simulink model "COM_ViconController_x4morf_quat"  (Simulink 8.6)
settings: Solver=FixedStepDiscrete  StartTime=0.0  StopTime=inf  FixedStep=ComMinSampleTime  RelTol=1e-3
values from neighbouring files (symbols this model uses):
  a_PWM = (MaxThrottle-MinThrottle)/(omega_r_max-omega_r_min)    [RobotParameters.m]
  b_PWM = MinThrottle - a_PWM*omega_r_min    [RobotParameters.m]
  BiasAcc = [0.52334832668 1 0]    [AccCalib_Transformation_GusRobot.mat]
  ComMinSampleTime = 1/400    (= 0.0025)    [init_ViconController_x4morf_quat.m]
  g = 9.81    [RobotParameters.m]    (also in init_ViconController_x4morf_quat.m)
  iGamma = inv(Gamma)    [RobotParameters.m]
  LandingHeight = 0.06    [init_ViconController_x4morf_quat.m]
  m = 0.376    [RobotParameters.m]
  MaxThrottle = 2000    [RobotParameters.m]
  MinThrottle = 1100    [RobotParameters.m]
  Tacc = [1  0  0; 0  1  0; 0  0  1]    [AccCalib_Transformation_GusRobot.mat]
  Tmax = .160    (= 0.16)    [RobotParameters.m]
  Tmin = .02    (= 0.02)    [RobotParameters.m]
  Velocity_0 = [Vx_0 Vy_0 Vz_0]    [RobotParameters.m]
undefined symbols (not defined in the file or in its folder): DiscIntNeverNeededParam, Gumstix, MPU6050, UAVstruct
undefined symbols (not defined in the file): AccMax, AccMin, b_est0, PositionMax, PositionMin, SpeedMax, SpeedMin, Ts_AttitudeLoop, Ts_Wifi
libraries: simulink x16, simulink_extras x6
(part 1 of 2)
settings Model: Creator=Kjenab  LastModifiedBy=valentin_riviere  ExtModeTrigDuration=10000
settings SolverCC: PositivePriorityOrder=on
settings DataIOCC: SaveFormat=StructureWithTime
settings OptimizationCC: InitFltsAndDblsToZero=on  OptimizeModelRefInitCode=on  LifeSpan=Inf  SimCompilerOptimization=on
settings DebuggingCC: SaveWithParameterizedLinksMsg=none  UnderspecifiedInitializationDetection=Simplified  MergeDetectMultiDrivingBlocksExec=error  FcnCallInpInsideContextMsg=UseLocalSettings
settings HardwareCC: ProdHWDeviceType=Generic->Unspecified (assume 32-bit Generic)
settings RTWCC: SystemTargetFile=ert.tlc  GenCodeOnly=on  GenerateMakefile=off  TemplateMakefile=ert_default_tmf  PostCodeGenCommand=packNGo(buildInfo, {'packType' 'hierarchical'})  Description=Embedded Coder  RTWCompilerOptimization=on
settings CodeAppCC: IgnoreCustomStorageClasses=off  CustomSymbolStrType=$N$R$M  InternalIdentifier=Classic
settings ERTTargetCC: MultiwordLength=2048  GenerateSampleERTMain=on  ERTCustomFileTemplate=example_file_process.tlc  ConvertIfToSwitch=off  SuppressUnreachableDefaultCases=off

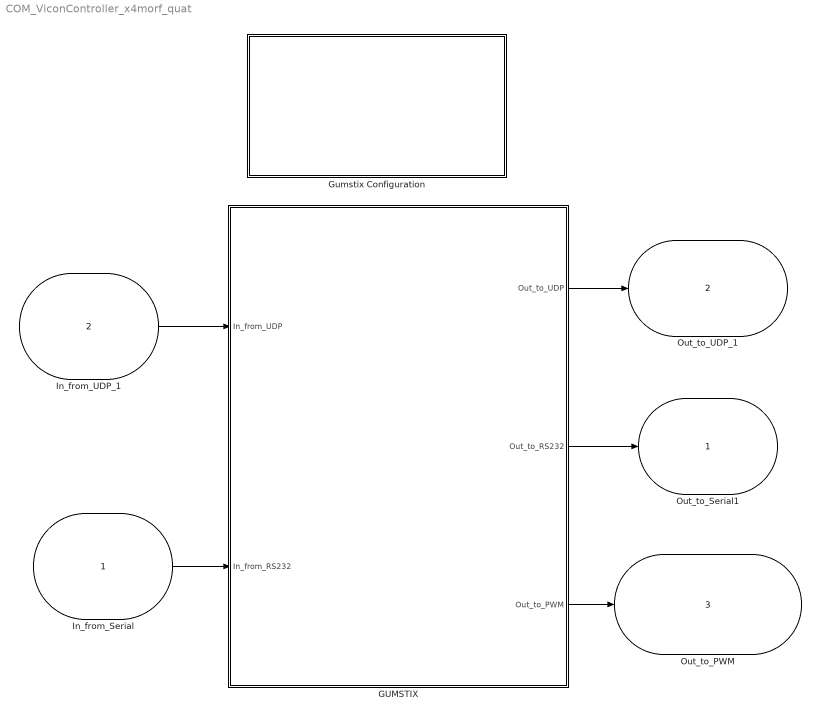
== system COM_ViconController_x4morf_quat ==
  In_from_Serial : Inport  OutDataTypeStr=int16  PortDimensions=Gumstix.RS232.Reception(1).NbData  SampleTime=Gumstix.RS232.Reception(1).SampleTime  mask{RS232_NbData=11, RS232_DataType=int16, RS232_Port=/dev/ttyO0, RS232_BaudRate=115200, RS232_SampleTime=Ts_AttitudeLoop, RS232_BlockingReception=OFF (try to read the n data), RS232_BlockingTimeOut=0.00022, RS232_StreamHeaderReception=1 byte, RS232_StreamHeaderValue=170, RS232_StartProtocol=SendStart -> WaitStart, RS232_StartTimeOut=100, RS232_StartStream=START, RS232_StopProtocol=None, RS232_StopTimeOut=100, RS232_StopStream=STOP}
      mask prompts: RS232_NbData "Number of Received Data"; RS232_DataType "RS232 Data Type"; RS232_Port "Serial Port"; RS232_BaudRate "BaudRate"; RS232_SampleTime "Reception Sample Time [s]"; RS232_BlockingReception "Blocking Reception"; RS232_BlockingTimeOut "Blocking Time Out [s]"; RS232_StreamHeaderReception "Stream Header"; RS232_StreamHeaderValue "Stream header value [0-255]"; RS232_StartProtocol "START Protocols"; RS232_StartTimeOut "Start Stream Waiting TimeOut [ms]"; RS232_StartStream "Start Message"; RS232_StopProtocol "STOP Protocols"; RS232_StopTimeOut "Stop Stream Waiting TimeOut [ms]"; RS232_StopStream "Stop Message"
      mask init:
      | for i=1:1:15
      |     ProcessRS232InportMask_COM(gcb, i);
      | end
      mask Callback RS232_NbData: ProcessRS232InportMask_COM(gcb, 1);
      mask TypeOptions RS232_DataType: double64 | float32 | int32 | unsigned int32 | int16 | unsigned int16 | char8 | unsigned char8
      mask Callback RS232_DataType: ProcessRS232InportMask_COM(gcb, 2);
      mask TypeOptions RS232_Port: /dev/ttyO0 | /dev/ttyO1 | /dev/ttyO2 | /dev/ttyO3 | /dev/ttyO4 | /dev/ttyO5 | /dev/ttyO6 | /dev/ttyO7 | /dev/ttyO8 | /dev/ttyO9 | /dev/ttyO10 | /dev/ttyO11 | /dev/ttyO12 | /dev/ttyO13 | /dev/ttyO14 | /dev/ttyO15 | /dev/ttyUSB0 | /dev/ttyUSB1
      mask Callback RS232_Port: ProcessRS232InportMask_COM(gcb, 3);
      mask TypeOptions RS232_BaudRate: 50 | 75 | 110 | 134 | 150 | 200 | 300 | 600 | 1200 | 1800 | 2400 | 4800 | 9600 | 19200 | 38400 | 57600 | 115200 | 230400 | 460800 | 576000 | 921600 | 1000000 | 1152000 | 1500000 | 2000000 | 2500000 | 3000000 | 3500000 | 4000000
      mask Callback RS232_BaudRate: ProcessRS232InportMask_COM(gcb, 4);
      mask Callback RS232_SampleTime: ProcessRS232InportMask_COM(gcb, 5);
      mask TypeOptions RS232_BlockingReception: ON (wait the n data) | OFF (try to read the n data)
      mask Callback RS232_BlockingReception: ProcessRS232InportMask_COM(gcb, 6);
      mask Callback RS232_BlockingTimeOut: ProcessRS232InportMask_COM(gcb, 7);
      mask TypeOptions RS232_StreamHeaderReception: None | 1 byte
      mask Callback RS232_StreamHeaderReception: ProcessRS232InportMask_COM(gcb, 8);
      mask Callback RS232_StreamHeaderValue: ProcessRS232InportMask_COM(gcb, 9);
      mask TypeOptions RS232_StartProtocol: WaitStart -> SendStart | SendStart -> WaitStart | None
      mask Callback RS232_StartProtocol: ProcessRS232InportMask_COM(gcb, 10);
      mask Callback RS232_StartTimeOut: ProcessRS232InportMask_COM(gcb, 11);
      mask Callback RS232_StartStream: ProcessRS232InportMask_COM(gcb, 12);
      mask TypeOptions RS232_StopProtocol: WaitStop -> SendStop | SendStop -> WaitStop | None
      mask Callback RS232_StopProtocol: ProcessRS232InportMask_COM(gcb, 13);
      mask Callback RS232_StopTimeOut: ProcessRS232InportMask_COM(gcb, 14);
      mask Callback RS232_StopStream: ProcessRS232InportMask_COM(gcb, 15);
      mask Display: Display_RS232_Reception_Block;
  In_from_UDP_1 : Inport  Port=2  OutDataTypeStr=single  PortDimensions=Gumstix.UDP.Reception(1).NbData  SampleTime=Gumstix.UDP.Reception(1).SampleTime  mask{UDP_NbData=40, UDP_DataType=float32, UDP_remoteIPaddress='192.168.137.1', UDP_remotePort=2011, UDP_Interface=wlan0, UDP_localPort=2011, UDP_SampleTime=Ts_Wifi, UDP_BlockingReception=OFF (try to read the n data), UDP_BlockingTimeOut=0.1}
      mask prompts: UDP_NbData "Number of Received Data"; UDP_DataType "UDP Data Type"; UDP_remoteIPaddress "Remote peer's IP address (IPv4)"; UDP_remotePort "Remote peer's Port (1023<port<65536)"; UDP_Interface "Local Interface to use"; UDP_localPort "Local Port (1023<port<65536)"; UDP_SampleTime "Reception Sample Time [s]"; UDP_BlockingReception "Blocking Reception"; UDP_BlockingTimeOut "Blocking Time Out [s]"
      mask init:
      | for i=1:1:8
      |     ProcessUDPInportMask_COM(gcb, i);
      | end
      mask Callback UDP_NbData: ProcessUDPInportMask_COM(gcb, 1);
      mask TypeOptions UDP_DataType: double64 | float32 | int32 | unsigned int32 | int16 | unsigned int16 | char8 | unsigned char8
      mask Callback UDP_DataType: ProcessUDPInportMask_COM(gcb, 2);
      mask Callback UDP_remoteIPaddress: ProcessUDPInportMask_COM(gcb, 3);
      mask Callback UDP_remotePort: ProcessUDPInportMask_COM(gcb, 4);
      mask TypeOptions UDP_Interface: wlan0 | eth0
      mask Callback UDP_Interface: ProcessUDPInportMask_COM(gcb, 5);
      mask Callback UDP_localPort: ProcessUDPInportMask_COM(gcb, 6);
      mask Callback UDP_SampleTime: ProcessUDPInportMask_COM(gcb, 7);
      mask TypeOptions UDP_BlockingReception: ON (wait the n data until the Time Out) | OFF (try to read the n data)
      mask Callback UDP_BlockingReception: ProcessUDPInportMask_COM(gcb, 8);
      mask Callback UDP_BlockingTimeOut: ProcessUDPInportMask_COM(gcb, 9);
      mask Display: Display_UDP_Reception_Block;
  GUMSTIX : Subsystem
  Gumstix Configuration : Subsystem  mask{TimeSynchro=Internal Clock, RS232_InterruptSource=/dev/ttyO0, UDP_InterruptSource=wlan0, PrintfMode=off, FprintfMode=off, TimeLoggerMode=off, PrintfTimeMode=off, FprintfTimeMode=off, TaskingMode=Multi-Tasking, SchedPolicy=SCHED_FIFO     (Real-Time Scheduler), MaxTaskPriority=95, RTsystem=PREEMPT-RT, TargetEndianess=Unspecified (default), TargetWordSize=32 bits (default)}
      mask prompts: TimeSynchro "Time Scheduler"; RS232_InterruptSource "RS232 Interrupt Source"; UDP_InterruptSource "UDP Interrupt Source"; PrintfMode "Verbose mode activated in the Gumstix console"; FprintfMode "Verbose mode logged in a file (onto Gumstix)"; TimeLoggerMode "Time logger mode activated (log time exec of each task)"; PrintfTimeMode "Execution time plotted in the Gumstix console"; FprintfTimeMode "Execution time logged in a file (onto Gumstix)"; TaskingMode "Tasking Mode"; SchedPolicy "Scheduler Policy"; MaxTaskPriority "Maximum Task Priority [1-99]"; RTsystem "RT system"; TargetEndianess "Target Endianess"; TargetWordSize "Target Word Size"
      mask init:
      | for i=1:1:14
      |     ProcessConfigMask_COM(gcb, i);
      | end
      mask TypeOptions TimeSynchro: RS232 Reception | Internal Clock | UDP Reception
      mask Callback TimeSynchro: ProcessConfigMask_COM(gcb, 1);
      mask TypeOptions RS232_InterruptSource: /dev/ttyS0 | /dev/ttyS1 | /dev/ttyS2 | /dev/ttyS3 | /dev/ttyO0 | /dev/ttyO1 | /dev/ttyO2 | /dev/ttyO3
      mask Callback RS232_InterruptSource: ProcessConfigMask_COM(gcb, 2);
      mask TypeOptions UDP_InterruptSource: wlan0 | eth0
      mask Callback UDP_InterruptSource: ProcessConfigMask_COM(gcb, 3);
      mask TypeOptions PrintfMode: off | on
      mask Callback PrintfMode: ProcessConfigMask_COM(gcb, 4);
      mask TypeOptions FprintfMode: off | on
      mask Callback FprintfMode: ProcessConfigMask_COM(gcb, 5);
      mask TypeOptions TimeLoggerMode: off | on
      mask Callback TimeLoggerMode: ProcessConfigMask_COM(gcb, 6);
      mask TypeOptions PrintfTimeMode: off | on
      mask Callback PrintfTimeMode: ProcessConfigMask_COM(gcb, 7);
      mask TypeOptions FprintfTimeMode: off | on
      mask Callback FprintfTimeMode: ProcessConfigMask_COM(gcb, 8);
      mask TypeOptions TaskingMode: Multi-Tasking | Single-Tasking
      mask Callback TaskingMode: ProcessConfigMask_COM(gcb, 9);
      mask TypeOptions SchedPolicy: SCHED_FIFO     (Real-Time Scheduler) | SCHED_RR        (Real-Time Scheduler) | SCHED_OTHER (NO Real-Time Scheduler)
      mask Callback SchedPolicy: ProcessConfigMask_COM(gcb, 10);
      mask Callback MaxTaskPriority: ProcessConfigMask_COM(gcb, 11);
      mask TypeOptions RTsystem: PREEMPT-RT | XENOMAI
      mask Callback RTsystem: ProcessConfigMask_COM(gcb, 12);
      mask TypeOptions TargetEndianess: Unspecified (default) | Little-Endian | Big-Endian
      mask Callback TargetEndianess: ProcessConfigMask_COM(gcb, 13);
      mask TypeOptions TargetWordSize: 32 bits (default) | 64 bits (LLP64) | 64 bits (LP64)
      mask Callback TargetWordSize: ProcessConfigMask_COM(gcb, 14);
      mask Display: image(imread('Configuration_v2.jpg'));
  Out_to_Serial1 : Outport  OutDataTypeStr=int16  PortDimensions=Gumstix.RS232.Emission(1).NbData  SampleTime=Gumstix.RS232.Emission(1).SampleTime  mask{RS232_NbData=4, RS232_DataType=int16, RS232_Port=/dev/ttyO0, RS232_BaudRate=115200, RS232_SampleTime=Ts_AttitudeLoop, RS232_StreamHeaderReception=1 byte, RS232_StreamHeaderValue=170, RS232_StartProtocol=SendStart -> WaitStart, RS232_StartTimeOut=100, RS232_StartStream=START, RS232_StopProtocol=None, RS232_StopTimeOut=100, RS232_StopStream=STOP}
      mask prompts: RS232_NbData "Number of Sent Data"; RS232_DataType "RS232 Data Type"; RS232_Port "Serial Port"; RS232_BaudRate "BaudRate"; RS232_SampleTime "Sample Time [s]"; RS232_StreamHeaderReception "Stream Header"; RS232_StreamHeaderValue "Stream header value [0-255]"; RS232_StartProtocol "RS232 Start Protocol"; RS232_StartTimeOut "Start Stream Waiting TimeOut [ms]"; RS232_StartStream "Start Message"; RS232_StopProtocol "RS232 Stop Protocol"; RS232_StopTimeOut "Stop Stream Waiting TimeOut [ms]"; RS232_StopStream "Stop Message"
      mask init:
      | for i=1:1:13
      |     ProcessRS232OutportMask_COM(gcb, i);
      | end
      mask Callback RS232_NbData: ProcessRS232OutportMask_COM(gcb, 1);
      mask TypeOptions RS232_DataType: double64 | float32 | int32 | unsigned int32 | int16 | unsigned int16 | char8 | unsigned char8
      mask Callback RS232_DataType: ProcessRS232OutportMask_COM(gcb, 2);
      mask TypeOptions RS232_Port: /dev/ttyO0 | /dev/ttyO1 | /dev/ttyO2 | /dev/ttyO3 | /dev/ttyO4 | /dev/ttyO5 | /dev/ttyO6 | /dev/ttyO7 | /dev/ttyO8 | /dev/ttyO9 | /dev/ttyO10 | /dev/ttyO11 | /dev/ttyO12 | /dev/ttyO13 | /dev/ttyO14 | /dev/ttyO15 | /dev/ttyUSB0 | /dev/ttyUSB1
      mask Callback RS232_Port: ProcessRS232OutportMask_COM(gcb, 3);
      mask TypeOptions RS232_BaudRate: 50 | 75 | 110 | 134 | 150 | 200 | 300 | 600 | 1200 | 1800 | 2400 | 4800 | 9600 | 19200 | 38400 | 57600 | 115200 | 230400 | 460800 | 576000 | 921600 | 1000000 | 1152000 | 1500000 | 2000000 | 2500000 | 3000000 | 3500000 | 4000000
      mask Callback RS232_BaudRate: ProcessRS232OutportMask_COM(gcb, 4);
      mask Callback RS232_SampleTime: ProcessRS232OutportMask_COM(gcb, 5);
      mask TypeOptions RS232_StreamHeaderReception: None | 1 byte
      mask Callback RS232_StreamHeaderReception: ProcessRS232OutportMask_COM(gcb, 6);
      mask Callback RS232_StreamHeaderValue: ProcessRS232OutportMask_COM(gcb, 7);
      mask TypeOptions RS232_StartProtocol: WaitStart -> SendStart | SendStart -> WaitStart | None
      mask Callback RS232_StartProtocol: ProcessRS232OutportMask_COM(gcb, 8);
      mask Callback RS232_StartTimeOut: ProcessRS232OutportMask_COM(gcb, 9);
      mask Callback RS232_StartStream: ProcessRS232OutportMask_COM(gcb, 10);
      mask TypeOptions RS232_StopProtocol: WaitStop -> SendStop | SendStop -> WaitStop | None
      mask Callback RS232_StopProtocol: ProcessRS232OutportMask_COM(gcb, 11);
      mask Callback RS232_StopTimeOut: ProcessRS232OutportMask_COM(gcb, 12);
      mask Callback RS232_StopStream: ProcessRS232OutportMask_COM(gcb, 13);
      mask Display: Display_RS232_Emission_Block;
  Out_to_UDP_1 : Outport  Port=2  OutDataTypeStr=single  PortDimensions=Gumstix.UDP.Emission(1).NbData  SampleTime=Gumstix.UDP.Emission(1).SampleTime  mask{UDP_NbData=69, UDP_DataType=float32, UDP_RemoteIPaddress='192.168.137.1', UDP_RemotePort=2011, UDP_Interface=wlan0, UDP_LocalPort=2011, UDP_SampleTime=Ts_Wifi}
      mask prompts: UDP_NbData "Number of Sent Data"; UDP_DataType "UDP Data Type"; UDP_RemoteIPaddress "remote peer's IP address (IPv4)"; UDP_RemotePort "remote peer's Port (1023<port<65536)"; UDP_Interface "Local Interface to use for UDP"; UDP_LocalPort "Local port to use"; UDP_SampleTime "Emission Sample Time [s]"
      mask init:
      | for i=1:1:7
      |     ProcessUDPOutportMask_COM(gcb, i);
      | end
      mask Callback UDP_NbData: ProcessUDPOutportMask_COM(gcb, 1);
      mask TypeOptions UDP_DataType: double64 | float32 | int32 | unsigned int32 | int16 | unsigned int16 | char8 | unsigned char8
      mask Callback UDP_DataType: ProcessUDPOutportMask_COM(gcb, 2);
      mask Callback UDP_RemoteIPaddress: ProcessUDPOutportMask_COM(gcb, 3);
      mask Callback UDP_RemotePort: ProcessUDPOutportMask_COM(gcb, 4);
      mask TypeOptions UDP_Interface: wlan0 | eth0
      mask Callback UDP_Interface: ProcessUDPOutportMask_COM(gcb, 5);
      mask Callback UDP_LocalPort: ProcessUDPOutportMask_COM(gcb, 6);
      mask Callback UDP_SampleTime: ProcessUDPOutportMask_COM(gcb, 7);
      mask Display: Display_UDP_Emission_Block;
  Out_to_PWM : Outport  Port=3  OutDataTypeStr=uint16  PortDimensions=evalin('base', 'length(Gumstix.PWM.ActivePwm)')  SampleTime=evalin('base', 'Gumstix.PWM.SampleTime')  mask{TimersList=10, PwmFrequency=333, PwmMode=DUTY_CYCLE Mode, ServoMin=10000, ServoMax=20000, PWM_DefaultValue=30, PWM_SampleTime=ComMinSampleTime*3, PWM_KeepAfterStop=on}
      mask prompts: TimersList "Active PWM (example: [8,9,10,11])"; PwmFrequency "PWM Frequency [Hz]"; PwmMode "PWM Mode"; ServoMin "Servo Min Value [tenth's of us]"; ServoMax "Servo Max Value [tenth's of us]"; PWM_DefaultValue "Default Pwm Value"; PWM_SampleTime "Refresh Sample Time [s]"; PWM_KeepAfterStop "Keep Default Pwm Value after program stop"
      mask init:
      | for i=1:1:8
      |     ProcessPWMmask_COM(gcb, i);
      | end
      mask Callback TimersList: ProcessPWMmask_COM(gcb, 1);
      mask Callback PwmFrequency: ProcessPWMmask_COM(gcb, 2);
      mask TypeOptions PwmMode: SERVO Mode | DUTY_CYCLE Mode
      mask Callback PwmMode: ProcessPWMmask_COM(gcb, 3);
      mask Callback ServoMin: ProcessPWMmask_COM(gcb, 4);
      mask Callback ServoMax: ProcessPWMmask_COM(gcb, 5);
      mask Callback PWM_DefaultValue: ProcessPWMmask_COM(gcb, 6);
      mask Callback PWM_SampleTime: ProcessPWMmask_COM(gcb, 7);
      mask Callback PWM_KeepAfterStop: ProcessPWMmask_COM(gcb, 8);
      mask Display: Display_PWM_Block;
  wires:
  In_from_UDP_1/1 -> GUMSTIX/1(In_from_UDP)
  In_from_Serial/1 -> GUMSTIX/2(In_from_RS232)
  GUMSTIX/1(Out_to_UDP) -> Out_to_UDP_1/1
  GUMSTIX/2(Out_to_RS232) -> Out_to_Serial1/1
  GUMSTIX/3(Out_to_PWM) -> Out_to_PWM/1

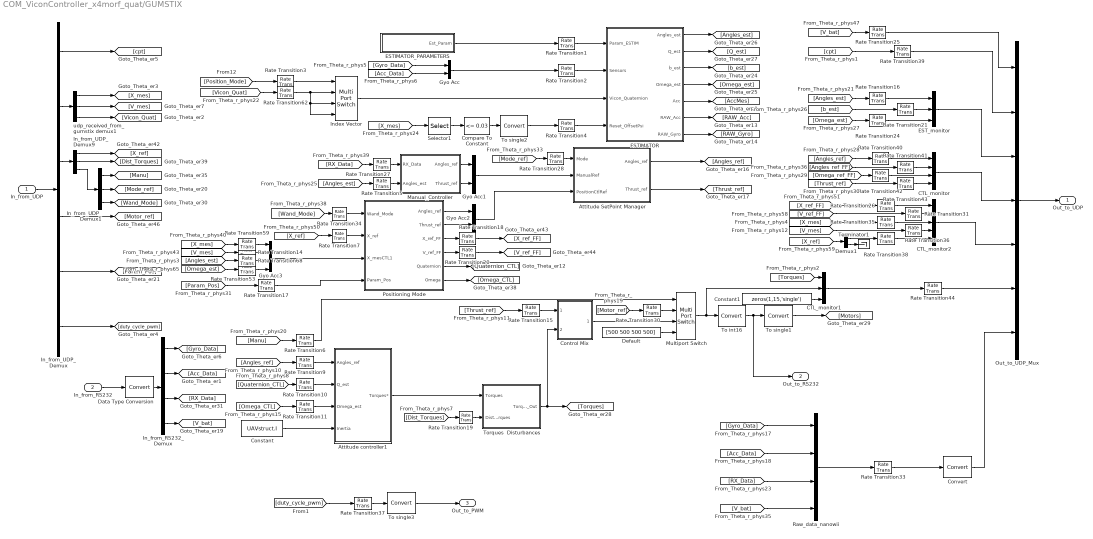
== system COM_ViconController_x4morf_quat/GUMSTIX ==
  In_from_UDP : Inport
  In_from_RS232 : Inport  Port=2
  Attitude controller1 : Subsystem
  Attitude SetPoint Manager : Subsystem
  CTL_monitor : Mux  Inputs=[3 3 3 1]
  CTL_monitor1 : Mux  Inputs=[3 4 15]
  CTL_monitor2 : Mux  Inputs=[3 3 3 3 3]
  Compare To Constant : simulink/Logic and Bit Operations/Compare To Constant  relop=<=  const=0.03  OutDataTypeStr=uint8
  Constant : Constant  Value=UAVstruct.I
  Constant1 : Constant  Value=zeros(1,15,'single')
  Control Mix : Subsystem
  Convert : DataTypeConversion  RndMeth=Nearest
  Data Type Conversion : DataTypeConversion
  Default : Constant  Value=[500 500 500 500]  OutDataTypeStr=Inherit: Inherit via back propagation  SampleTime=-1
  Demux1 : Demux  Outputs=[3 1]
  ESTIMATOR : Subsystem
  ESTIMATOR_PARAMETERS : Subsystem
  EST_monitor : Mux  Inputs=[3 3 3]
  Gyo Acc : Mux  Inputs=2
  Gyo Acc1 : Mux  Inputs=2
  Gyo Acc2 : Mux  Inputs=2
  Gyo Acc3 : Mux  Inputs=[3; 3; 3; 3]
  In_from_RS232_Demux : Demux  Outputs=[3 3 4 1]
  In_from_UDP_Demux : Demux  Outputs=[1 10 12 4 12 1]
  In_from_UDP_Demux1 : Demux  Outputs=3
  In_from_UDP_Demux9 : Demux  Outputs=[4 5 3]
  Index Vector : MultiPortSwitch  Inputs=2  DataPortForDefault=Additional data port  DiagnosticForDefault=None
  Manual_Controller : Subsystem
  Multiport Switch : MultiPortSwitch  Inputs=2  DataPortForDefault=Additional data port  DiagnosticForDefault=None
  Out_to_UDP_Mux : Mux  Inputs=[1 1 9 10 15 22 11]
  Positioning Mode : Subsystem
  Rate Transition{1..4,6,9..11,15,19,30,62} (12 alike) : RateTransition  Deterministic=off  OutPortSampleTime=Ts_AttitudeLoop
  Rate Transition{14,16,18,20..21,24..26,31,33,35..44,53,59,68} (23 alike) : RateTransition  Deterministic=off
  Rate Transition{5,7,17,27..28,34} (6 alike) : RateTransition  Deterministic=off  OutPortSampleTime=Ts_PositionLoop
  Raw_data_nanowii : Mux  Inputs=[3 3 4 1]
  Selector1 : Selector  InputPortWidth=3  IndexOptions=Index vector (dialog)  Indices=[3]  OutputSizes=1
  Terminator1 : Terminator
  To int16 : DataTypeConversion  RndMeth=Nearest
  To single1 : DataTypeConversion  RndMeth=Nearest
  To single2 : DataTypeConversion  RndMeth=Nearest
  To single3 : DataTypeConversion  RndMeth=Nearest
  Torques  Disturbances : Subsystem
  udp_received_from_gumstix demux1 : Demux  Outputs=[3 3 4]
  Out_to_UDP : Outport
  Out_to_RS232 : Outport  Port=2
  Out_to_PWM : Outport  Port=3
  wires:
  Out_to_UDP_Mux/1 -> Out_to_UDP/1
  In_from_RS232/1 -> Data Type Conversion/1
  In_from_UDP/1 -> In_from_UDP_Demux/1
  In_from_RS232_Demux/1 -> [Gyro_Data]
  Data Type Conversion/1 -> In_from_RS232_Demux/1
  [Gyro_Data] -> Gyo Acc/1
  [Acc_Data] -> Gyo Acc/2
  [Thrust_ref] -> Rate Transition15/1
  [Manu] -> Rate Transition6/1
  [Motor_ref] -> Rate Transition30/1
  In_from_UDP_Demux/1 -> [cpt]
  [Angles_ref] -> Rate Transition9/1
  Gyo Acc/1 -> Rate Transition2/1
  ESTIMATOR/1(Angles_est) -> [Angles_est]
  ESTIMATOR/2(Q_est) -> [Q_est]
  ESTIMATOR/3(b_est) -> [b_est]
  [Omega_CTL] -> Rate Transition11/1
  Control Mix/1(PWM_sat) -> Multiport Switch/3
  [Angles_ref] -> Rate Transition40/1
  To single1/1 -> [Motors]
  [Angles_est] -> Rate Transition16/1
  [b_est] -> Rate Transition21/1
  [Omega_est] -> Rate Transition24/1
  Multiport Switch/1 -> To int16/1, CTL_monitor1/2
  [RX_Data] -> Rate Transition27/1
  In_from_UDP_Demux1/1 -> [Manu]
  In_from_UDP_Demux1/2 -> [Mode_ref]
  [V_bat] -> Rate Transition25/1
  [Quaternion_CTL] -> Rate Transition10/1
  To int16/1 -> To single1/1, Out_to_RS232/1
  [X_ref_FF] -> Rate Transition26/1
  [V_mes] -> Rate Transition36/1
  [X_mes] -> Rate Transition35/1
  [V_ref_FF] -> Rate Transition31/1
  Demux1/1 -> Rate Transition38/1
  [X_ref] -> Demux1/1
  Demux1/2 -> Terminator1/1
  [cpt] -> Rate Transition39/1
  Default/1 -> Multiport Switch/4
  [X_mes] -> Selector1/1
  Selector1/1 -> Compare To Constant/1
  Compare To Constant/1 -> To single2/1
  [Angles_est] -> Rate Transition5/1
  Rate Transition5/1 -> Manual_Controller/2(Angles_est)
  [Torques] -> CTL_monitor1/1
  Torques  Disturbances/1(Torques_Out) -> Control Mix/2(Torques), [Torques]
  [Thrust_ref] -> Rate Transition43/1
  [Omega_ref_FF] -> Rate Transition42/1
  [Angles_ref_FF] -> Rate Transition41/1
  ESTIMATOR_PARAMETERS/1(Est_Param) -> Rate Transition1/1
  In_from_UDP_Demux1/3 -> [Wand_Mode]
  In_from_RS232_Demux/2 -> [Acc_Data]
  In_from_RS232_Demux/3 -> [RX_Data]
  [X_ref] -> Rate Transition7/1
  [Angles_est] -> Rate Transition68/1
  [Param_Pos] -> Rate Transition17/1
  [Wand_Mode] -> Rate Transition34/1
  Positioning Mode/4(V_ref_FF) -> Rate Transition20/1
  Positioning Mode/3(X_ref_FF) -> Rate Transition18/1
  Manual_Controller/1(Angles_ref) -> Gyo Acc1/1
  Manual_Controller/2(Thrust_ref) -> Gyo Acc1/2
  Positioning Mode/1(Angles_ref) -> Gyo Acc2/1
  Positioning Mode/2(Thrust_ref) -> Gyo Acc2/2
  Gyo Acc2/1 -> Attitude SetPoint Manager/3(PositionCtlRef)
  Gyo Acc1/1 -> Attitude SetPoint Manager/2(ManualRef)
  [Mode_ref] -> Rate Transition28/1
  Attitude SetPoint Manager/1(Angles_ref) -> [Angles_ref]
  Attitude SetPoint Manager/2(Thrust_ref) -> [Thrust_ref]
  ESTIMATOR/4(Omega_est) -> [Omega_est]
  [Dist_Torques] -> Rate Transition19/1
  udp_received_from_gumstix demux1/1 -> [X_mes]
  udp_received_from_gumstix demux1/2 -> [V_mes]
  Rate Transition18/1 -> [X_ref_FF]
  Rate Transition20/1 -> [V_ref_FF]
  Rate Transition27/1 -> Manual_Controller/1(RX_Data)
  Rate Transition28/1 -> Attitude SetPoint Manager/1(Mode)
  Rate Transition26/1 -> CTL_monitor2/1
  Rate Transition31/1 -> CTL_monitor2/2
  Rate Transition35/1 -> CTL_monitor2/3
  Rate Transition38/1 -> CTL_monitor2/5
  Rate Transition36/1 -> CTL_monitor2/4
  In_from_RS232_Demux/4 -> [V_bat]
  Rate Transition1/1 -> ESTIMATOR/1(Param_ESTIM)
  Rate Transition2/1 -> ESTIMATOR/2(Sensors)
  To single2/1 -> Rate Transition4/1
  Rate Transition4/1 -> ESTIMATOR/4(Reset_OffsetPsi)
  Rate Transition6/1 -> Multiport Switch/1
  Rate Transition9/1 -> Attitude controller1/1(Angles_ref)
  Rate Transition10/1 -> Attitude controller1/2(Q_est)
  Rate Transition11/1 -> Attitude controller1/3(Omega_est)
  Rate Transition15/1 -> Control Mix/1(Thrust)
  Rate Transition19/1 -> Torques  Disturbances/2(Dist_Torques)
  Rate Transition30/1 -> Multiport Switch/2
  Rate Transition16/1 -> EST_monitor/1
  Rate Transition21/1 -> EST_monitor/2
  Rate Transition24/1 -> EST_monitor/3
  Rate Transition40/1 -> CTL_monitor/1
  Rate Transition41/1 -> CTL_monitor/2
  Rate Transition42/1 -> CTL_monitor/3
  Rate Transition43/1 -> CTL_monitor/4
  ESTIMATOR/5(Acc) -> [AccMes]
  ESTIMATOR/6(RAW_Acc) -> [RAW_Acc]
  ESTIMATOR/7(RAW_Gyro) -> [RAW_Gyro]
  [X_mes] -> Rate Transition59/1
  [V_mes] -> Rate Transition14/1
  [Vicon_Quat] -> Rate Transition62/1
  Index Vector/1 -> ESTIMATOR/3(Vicon_Quaternion)
  [Position_Mode] -> Rate Transition3/1
  Rate Transition3/1 -> Index Vector/1
  Rate Transition62/1 -> Index Vector/2, Index Vector/4, Index Vector/3
  Rate Transition34/1 -> Positioning Mode/1(Wand_Mode)
  Rate Transition7/1 -> Positioning Mode/2(X_ref)
  Rate Transition17/1 -> Positioning Mode/4(Param_Pos)
  Gyo Acc3/1 -> Positioning Mode/3(X_mesCTL1)
  Rate Transition59/1 -> Gyo Acc3/1
  Rate Transition14/1 -> Gyo Acc3/2
  Rate Transition68/1 -> Gyo Acc3/3
  [Omega_est] -> Rate Transition53/1
  Positioning Mode/5(Quaternion) -> [Quaternion_CTL]
  Positioning Mode/6(Omega) -> [Omega_CTL]
  Rate Transition53/1 -> Gyo Acc3/4
  In_from_UDP_Demux9/1 -> [X_ref]
  In_from_UDP_Demux9/2 -> [Dist_Torques]
  In_from_UDP_Demux/5 -> [Param_Pos]
  [Gyro_Data] -> Raw_data_nanowii/1
  [Acc_Data] -> Raw_data_nanowii/2
  [RX_Data] -> Raw_data_nanowii/3
  [V_bat] -> Raw_data_nanowii/4
  Raw_data_nanowii/1 -> Rate Transition33/1
  Rate Transition33/1 -> Convert/1
  [duty_cycle_pwm] -> Rate Transition37/1
  Rate Transition37/1 -> To single3/1
  To single3/1 -> Out_to_PWM/1
  In_from_UDP_Demux/6 -> [duty_cycle_pwm]
  Constant/1 -> Attitude controller1/4(Inertia)
  CTL_monitor1/1 -> Rate Transition44/1
  Constant1/1 -> CTL_monitor1/3
  Attitude controller1/1(Torques*) -> Torques  Disturbances/1(Torques)
  In_from_UDP_Demux/4 -> [Motor_ref]
  In_from_UDP_Demux/2 -> udp_received_from_gumstix demux1/1
  udp_received_from_gumstix demux1/3 -> [Vicon_Quat]
  In_from_UDP_Demux/3 -> In_from_UDP_Demux9/1
  In_from_UDP_Demux9/3 -> In_from_UDP_Demux1/1
  Convert/1 -> Out_to_UDP_Mux/7
  Rate Transition44/1 -> Out_to_UDP_Mux/6
  CTL_monitor2/1 -> Out_to_UDP_Mux/5
  CTL_monitor/1 -> Out_to_UDP_Mux/4
  EST_monitor/1 -> Out_to_UDP_Mux/3
  Rate Transition39/1 -> Out_to_UDP_Mux/2
  Rate Transition25/1 -> Out_to_UDP_Mux/1

== system COM_ViconController_x4morf_quat/Gumstix Configuration ==

== system COM_ViconController_x4morf_quat/GUMSTIX/Attitude controller1 ==
  Angles_ref : Inport
  Q_est : Inport  Port=2
  Omega_est : Inport  Port=3
  Inertia : Inport  Port=4
  Attitude controller : Subsystem
  Rate Transition{1..4} (4 alike) : RateTransition  OutPortSampleTime=Ts_AttitudeLoop
  Terminator : Terminator
  Torques* : Outport
  wires:
  Angles_ref/1 -> Rate Transition3/1
  Q_est/1 -> Rate Transition1/1
  Inertia/1 -> Rate Transition2/1
  Attitude controller/1(Torques*) -> Torques*/1
  Omega_est/1 -> Rate Transition4/1
  Attitude controller/2(Omega_ref) -> Terminator/1
  Rate Transition3/1 -> Attitude controller/1(Angles_ref)
  Rate Transition2/1 -> Attitude controller/4(Inertia)
  Rate Transition1/1 -> Attitude controller/3(Q_hat)
  Rate Transition4/1 -> Attitude controller/2(Omega_est)

== system COM_ViconController_x4morf_quat/GUMSTIX/Attitude SetPoint Manager ==
  Mode : Inport
  ManualRef : Inport  Port=2
  PositionCtlRef : Inport  Port=3
  In_from_UDP_Demux2 : Demux  Outputs=[3 1]
  Manu_Ref : Constant  Value=[0; 0; 0; 0.3*m*g]  OutDataTypeStr=Inherit: Inherit via back propagation  SampleTime=-1
  Multiport Switch1 : MultiPortSwitch  DataPortForDefault=Additional data port  DiagnosticForDefault=None
  Angles_ref : Outport
  Thrust_ref : Outport  Port=2
  wires:
  Manu_Ref/1 -> Multiport Switch1/5, Multiport Switch1/2
  Mode/1 -> Multiport Switch1/1
  Multiport Switch1/1 -> In_from_UDP_Demux2/1
  In_from_UDP_Demux2/1 -> Angles_ref/1
  In_from_UDP_Demux2/2 -> Thrust_ref/1
  ManualRef/1 -> Multiport Switch1/4
  PositionCtlRef/1 -> Multiport Switch1/3

== system COM_ViconController_x4morf_quat/GUMSTIX/Control Mix ==
  Thrust : Inport
  Torques : Inport  Port=2
  Control_mix : Subsystem
  Omega_ref 2 PWM_ref : Subsystem
  Out_to_RS232_Mux : Mux
  Saturation MinThrottle MaxThrottle : Saturate  UpperLimit=MaxThrottle  LowerLimit=MinThrottle+20
  PWM_sat : Outport
  wires:
  Control_mix/1(omega_r1_ref) -> Out_to_RS232_Mux/1
  Control_mix/2(omega_r2_ref) -> Out_to_RS232_Mux/2
  Control_mix/3(omega_r3_ref) -> Out_to_RS232_Mux/3
  Control_mix/4(omega_r4_ref) -> Out_to_RS232_Mux/4
  Out_to_RS232_Mux/1 -> Omega_ref 2 PWM_ref/1(Omega_ref)
  Omega_ref 2 PWM_ref/1(PWM_ref) -> Saturation MinThrottle MaxThrottle/1
  Thrust/1 -> Control_mix/1(Thrust)
  Saturation MinThrottle MaxThrottle/1 -> PWM_sat/1
  Torques/1 -> Control_mix/2(Torques)

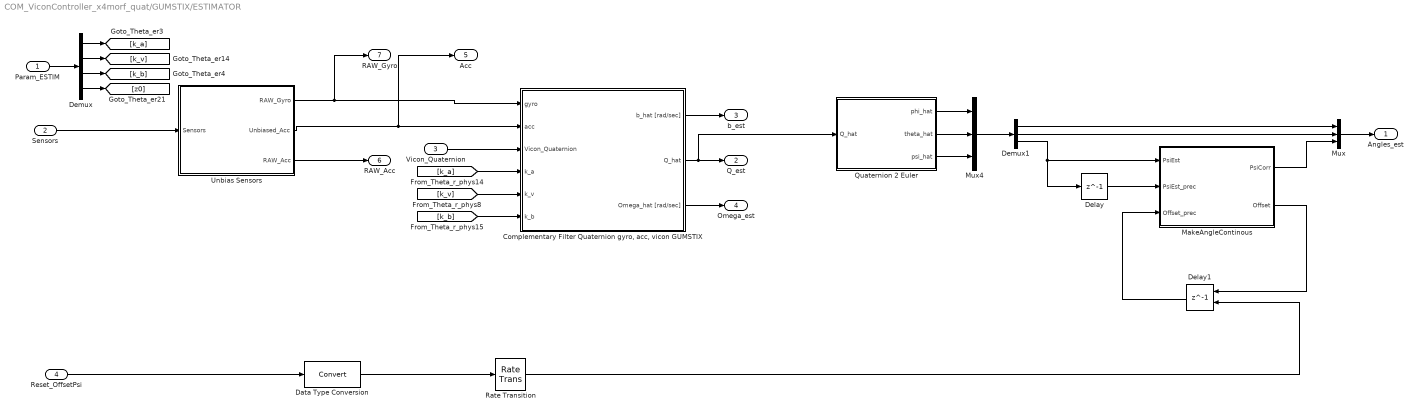
== system COM_ViconController_x4morf_quat/GUMSTIX/ESTIMATOR ==
  Param_ESTIM : Inport
  Sensors : Inport  Port=2
  Vicon_Quaternion : Inport  Port=3
  Reset_OffsetPsi : Inport  Port=4
  "Complementary Filter Quaternion gyro, acc, vicon GUMSTIX" : Subsystem  mask(COMPLEMENTARY FILTER){Ts_param=Ts_AttitudeLoop, b0_param=single(b_est0), Q0_param=single([1;0;0;0]), acc_ref_param=single([0;0;-g])}
      mask prompts: Ts_param "Sample Time [s]"; b0_param "Initial bias [deg/s]"; Q0_param "Initial Quaternion"; acc_ref_param "Accelerometer Reference"
      mask help:
      | This block assure a complementary filtering of IMU's data and vicon's data.
      |
      | ka: the gain to adjust accelerometer's sensibility
      |     A digonal matrix [3x3]:
      | kv: the gain to adjust vicon's sensibility
      |     A digonal matrix [3x3]
      | kb: the gain to adjust the bias sensibility
      |     A digonal matrix [3x3]
      |
      | Remark: For each diagonal matrix gain:
      |     - kx(1,1) = roll sensibilty
      |     - kx(2,2) = pitch sensibilty
      |     - kx(3,3) = yaw sensibilty
  Data Type Conversion : DataTypeConversion
  Delay : Delay  DelayLength=1
  Delay1 : Delay  DelayLength=1  ExternalReset=Level hold
      settings: InputPortMap=u0,r5
  Demux : Demux  Outputs=[3; 3; 3; 1]
  Demux1 : Demux  Outputs=3
  MakeAngleContinous : MATLAB Function  TreatAsAtomicUnit=on
  Mux : Mux  Inputs=3
  Mux4 : Mux  Inputs=3
  Quaternion 2 Euler : MATLAB Function  TreatAsAtomicUnit=on
  Rate Transition : RateTransition
  Unbias Sensors : Subsystem
  Angles_est : Outport
  Q_est : Outport  Port=2
  b_est : Outport  Port=3
  Omega_est : Outport  Port=4
  Acc : Outport  Port=5
  RAW_Acc : Outport  Port=6
  RAW_Gyro : Outport  Port=7
  wires:
  Sensors/1 -> Unbias Sensors/1(Sensors)
  Unbias Sensors/2(Unbiased_Acc) -> Acc/1, "Complementary Filter Quaternion gyro, acc, vicon GUMSTIX"/2(acc)
  Unbias Sensors/1(RAW_Gyro) -> "Complementary Filter Quaternion gyro, acc, vicon GUMSTIX"/1(gyro), RAW_Gyro/1
  "Complementary Filter Quaternion gyro, acc, vicon GUMSTIX"/1(b_hat [rad/sec]) -> b_est/1
  [k_a] -> "Complementary Filter Quaternion gyro, acc, vicon GUMSTIX"/4(k_a)
  "Complementary Filter Quaternion gyro, acc, vicon GUMSTIX"/2(Q_hat) -> Q_est/1, Quaternion 2 Euler/1(Q_hat)
  [k_v] -> "Complementary Filter Quaternion gyro, acc, vicon GUMSTIX"/5(k_v)
  [k_b] -> "Complementary Filter Quaternion gyro, acc, vicon GUMSTIX"/6(k_b)
  Param_ESTIM/1 -> Demux/1
  Demux/1 -> [k_a]
  Demux/2 -> [k_v]
  Demux/3 -> [k_b]
  Demux/4 -> [z0]
  Vicon_Quaternion/1 -> "Complementary Filter Quaternion gyro, acc, vicon GUMSTIX"/3(Vicon_Quaternion)
  Delay/1 -> MakeAngleContinous/2(PsiEst_prec)
  Delay1/1 -> MakeAngleContinous/3(Offset_prec)
  MakeAngleContinous/2(Offset) -> Delay1/1
  Mux/1 -> Angles_est/1
  Demux1/3 -> Delay/1, MakeAngleContinous/1(PsiEst)
  Demux1/2 -> Mux/2
  Demux1/1 -> Mux/1
  MakeAngleContinous/1(PsiCorr) -> Mux/3
  Reset_OffsetPsi/1 -> Data Type Conversion/1
  Rate Transition/1 -> Delay1/2
  Data Type Conversion/1 -> Rate Transition/1
  Unbias Sensors/3(RAW_Acc) -> RAW_Acc/1
  Quaternion 2 Euler/1(phi_hat) -> Mux4/1
  Quaternion 2 Euler/2(theta_hat) -> Mux4/2
  Quaternion 2 Euler/3(psi_hat) -> Mux4/3
  Mux4/1 -> Demux1/1
  "Complementary Filter Quaternion gyro, acc, vicon GUMSTIX"/3(Omega_hat [rad/sec]) -> Omega_est/1

== system COM_ViconController_x4morf_quat/GUMSTIX/ESTIMATOR_PARAMETERS ==
  Mux1 : Mux  Inputs=2
  Mux6 : Mux  Inputs=3
  Time Constant Gyro Filter : Constant  Value=0.3897 %exp(-2*pi*30*ComMinSampleTime)  OutDataTypeStr=Inherit: Inherit via back propagation  SampleTime=-1
  k_a : Constant  Value=[.4 .4 0]  OutDataTypeStr=Inherit: Inherit via back propagation  SampleTime=-1
  k_b : Constant  Value=[.08 .08 .08]  OutDataTypeStr=Inherit: Inherit via back propagation  SampleTime=-1
  k_v : Constant  Value=[0 0 2]  OutDataTypeStr=Inherit: Inherit via back propagation  SampleTime=-1
  Est_Param : Outport
  wires:
  k_a/1 -> Mux6/1
  k_b/1 -> Mux6/3
  k_v/1 -> Mux6/2
  Mux6/1 -> Mux1/1
  Time Constant Gyro Filter/1 -> Mux1/2
  Mux1/1 -> Est_Param/1

== system COM_ViconController_x4morf_quat/GUMSTIX/Manual_Controller ==
  RX_Data : Inport
  Angles_est : Inport  Port=2
  Gyo Acc2 : Mux  Inputs=[1 1 1]
  In_from_UDP_Demux1 : Demux  Outputs=3
  In_from_UDP_Demux3 : Demux  Outputs=[1 1 1 1]
  Product : Product  Inputs=*/  RndMeth=Zero
  Product1 : Product  Inputs=**  RndMeth=Zero
  RX Angles Ref  Generator : Subsystem
  Saturation1 : Saturate  UpperLimit=Tmax*9.81*4  LowerLimit=Tmin*9.81*4
  Terminator : Terminator
  Trigonometric Function : Trigonometry  Operator=cos
  Trigonometric Function1 : Trigonometry  Operator=cos
  Angles_ref : Outport
  Thrust_ref : Outport  Port=2
  wires:
  RX Angles Ref  Generator/1(Roll_ref) -> Gyo Acc2/1
  RX Angles Ref  Generator/2(Pitch_ref) -> Gyo Acc2/2
  RX Angles Ref  Generator/3(Yaw_ref) -> Gyo Acc2/3
  Angles_est/1 -> In_from_UDP_Demux1/1
  Product1/1 -> Product/2
  In_from_UDP_Demux1/1 -> Trigonometric Function/1
  In_from_UDP_Demux1/2 -> Trigonometric Function1/1
  In_from_UDP_Demux1/3 -> Terminator/1
  Trigonometric Function1/1 -> Product1/2
  Trigonometric Function/1 -> Product1/1
  RX Angles Ref  Generator/4(Throttle_ref) -> Product/1
  Product/1 -> Saturation1/1
  Saturation1/1 -> Thrust_ref/1
  In_from_UDP_Demux3/1 -> RX Angles Ref  Generator/1(Roll_RX)
  In_from_UDP_Demux3/2 -> RX Angles Ref  Generator/2(Pitch_RX)
  In_from_UDP_Demux3/3 -> RX Angles Ref  Generator/3(Yaw_RX)
  In_from_UDP_Demux3/4 -> RX Angles Ref  Generator/4(Throttle_RX)
  RX_Data/1 -> In_from_UDP_Demux3/1
  Gyo Acc2/1 -> Angles_ref/1

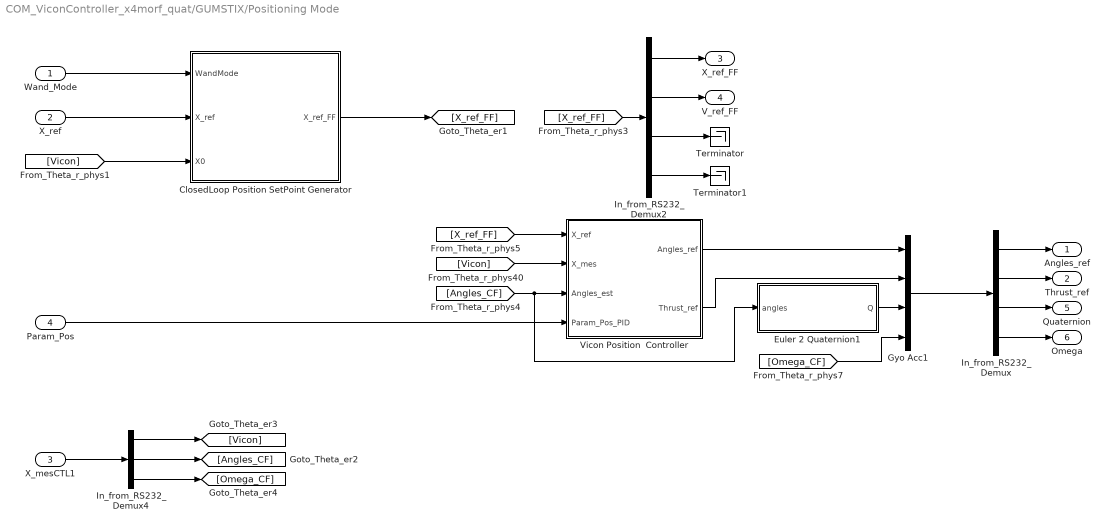
== system COM_ViconController_x4morf_quat/GUMSTIX/Positioning Mode ==
  Wand_Mode : Inport
  X_ref : Inport  Port=2
  X_mesCTL1 : Inport  Port=3
  Param_Pos : Inport  Port=4
  ClosedLoop Position SetPoint Generator : Subsystem
  Euler 2 Quaternion1 : MATLAB Function  TreatAsAtomicUnit=on
  Gyo Acc1 : Mux
  In_from_RS232_Demux : Demux  Outputs=[3 1 4 3]
  In_from_RS232_Demux2 : Demux  Outputs=[3 3 3 1]
  In_from_RS232_Demux4 : Demux  Outputs=[6 3 3]
  Terminator : Terminator
  Terminator1 : Terminator
  Vicon Position  Controller : Subsystem
  Angles_ref : Outport
  Thrust_ref : Outport  Port=2
  X_ref_FF : Outport  Port=3
  V_ref_FF : Outport  Port=4
  Quaternion : Outport  Port=5
  Omega : Outport  Port=6
  wires:
  [Vicon] -> Vicon Position  Controller/2(X_mes)
  Gyo Acc1/1 -> In_from_RS232_Demux/1
  In_from_RS232_Demux/1 -> Angles_ref/1
  In_from_RS232_Demux/2 -> Thrust_ref/1
  Wand_Mode/1 -> ClosedLoop Position SetPoint Generator/1(WandMode)
  [Vicon] -> ClosedLoop Position SetPoint Generator/3(X0)
  X_ref/1 -> ClosedLoop Position SetPoint Generator/2(X_ref)
  ClosedLoop Position SetPoint Generator/1(X_ref_FF) -> [X_ref_FF]
  [X_ref_FF] -> Vicon Position  Controller/1(X_ref)
  In_from_RS232_Demux2/1 -> X_ref_FF/1
  In_from_RS232_Demux2/2 -> V_ref_FF/1
  In_from_RS232_Demux2/3 -> Terminator/1
  In_from_RS232_Demux2/4 -> Terminator1/1
  [X_ref_FF] -> In_from_RS232_Demux2/1
  Vicon Position  Controller/1(Angles_ref) -> Gyo Acc1/1
  Vicon Position  Controller/2(Thrust_ref) -> Gyo Acc1/2
  X_mesCTL1/1 -> In_from_RS232_Demux4/1
  In_from_RS232_Demux4/1 -> [Vicon]
  In_from_RS232_Demux4/2 -> [Angles_CF]
  [Angles_CF] -> Vicon Position  Controller/3(Angles_est), Euler 2 Quaternion1/1(angles)
  Euler 2 Quaternion1/1(Q) -> Gyo Acc1/3
  [Omega_CF] -> Gyo Acc1/4
  In_from_RS232_Demux4/3 -> [Omega_CF]
  In_from_RS232_Demux/4 -> Omega/1
  In_from_RS232_Demux/3 -> Quaternion/1
  Param_Pos/1 -> Vicon Position  Controller/4(Param_Pos_PID)

== system COM_ViconController_x4morf_quat/GUMSTIX/Torques  Disturbances ==
  Torques : Inport
  Dist_Torques : Inport  Port=2
  Add : Sum
  Add1 : Sum
  Add2 : Sum
  Demux2 : Demux  Outputs=3
  Demux3 : Demux  Outputs=3
  Mux : Mux  Inputs=3
  Selector : Selector  InputPortWidth=5  IndexOptions=Index vector (dialog)  Indices=[1 2 3]  OutputSizes=1
  Selector2 : Selector  InputPortWidth=5  IndexOptions=Index vector (dialog)  Indices=4  OutputSizes=1
  Selector3 : Selector  InputPortWidth=5  IndexOptions=Index vector (dialog)  Indices=5  OutputSizes=1
  Triggered Subsystem : Subsystem  TreatAsAtomicUnit=on
  Torques_Out : Outport
  wires:
  Dist_Torques/1 -> Selector/1, Selector2/1, Selector3/1
  Selector/1 -> Triggered Subsystem/1(TorquesDist Mag)
  Selector3/1 -> Triggered Subsystem/Enable
  Demux2/1 -> Add/1
  Demux2/2 -> Add1/1
  Demux2/3 -> Add2/1
  Add/1 -> Mux/1
  Add1/1 -> Mux/2
  Add2/1 -> Mux/3
  Triggered Subsystem/1(DisturbTorques) -> Demux3/1
  Demux3/2 -> Add1/2
  Demux3/1 -> Add/2
  Demux3/3 -> Add2/2
  Selector2/1 -> Triggered Subsystem/2(Dt)
  Torques/1 -> Demux2/1
  Mux/1 -> Torques_Out/1

== system COM_ViconController_x4morf_quat/GUMSTIX/Attitude controller1/Attitude controller ==
  Angles_ref : Inport
  Omega_est : Inport  Port=2
  Q_hat : Inport  Port=3
  Inertia : Inport  Port=4
  3rd order filter : Subsystem
  Attitude Controller : MATLAB Function  TreatAsAtomicUnit=on
  Euler 2 Quaternion : MATLAB Function  TreatAsAtomicUnit=on
  Terminator : Terminator
  Terminator1 : Terminator
  derivation : Subsystem
  derivation1 : Subsystem
  kO : Constant  Value=[20 20 20]'
  kR : Constant  Value=[200 200 200]'
  Torques* : Outport
  Omega_ref : Outport  Port=2
  wires:
  Euler 2 Quaternion/1(Q) -> Attitude Controller/1(Q_ref)
  Q_hat/1 -> Attitude Controller/2(Q_est)
  derivation/1(Out) -> Attitude Controller/3(Omega_ref), derivation1/1(In), Omega_ref/1
  derivation1/1(Out) -> Attitude Controller/5(dOmega_ref)
  kR/1 -> Attitude Controller/7(kR)
  kO/1 -> Attitude Controller/8(kO)
  Omega_est/1 -> Attitude Controller/4(Omega_est)
  Angles_ref/1 -> 3rd order filter/1(In1)
  3rd order filter/1(Out1) -> derivation/1(In), Euler 2 Quaternion/1(angles)
  Attitude Controller/1(Torques) -> Torques*/1
  Inertia/1 -> Attitude Controller/6(I)
  Attitude Controller/2(eR) -> Terminator/1
  Attitude Controller/3(eO) -> Terminator1/1

== system COM_ViconController_x4morf_quat/GUMSTIX/Control Mix/Control_mix ==
  Thrust : Inport
  Torques : Inport  Port=2
  Demux : Demux
  Gain : Gain  Gain=iGamma  Multiplication=Matrix(K*u)
  Mux : Mux  Inputs=2
  Rate Transition : RateTransition
  Saturation : Saturate  UpperLimit=inf  LowerLimit=0
  Sqrt : Sqrt  SaturateOnIntegerOverflow=on
  omega_r1_ref : Outport
  omega_r2_ref : Outport  Port=2
  omega_r3_ref : Outport  Port=3
  omega_r4_ref : Outport  Port=4
  wires:
  Thrust/1 -> Mux/1
  Torques/1 -> Mux/2
  Mux/1 -> Gain/1
  Gain/1 -> Saturation/1
  Demux/1 -> omega_r1_ref/1
  Demux/2 -> omega_r2_ref/1
  Demux/3 -> omega_r3_ref/1
  Demux/4 -> omega_r4_ref/1
  Sqrt/1 -> Rate Transition/1
  Saturation/1 -> Sqrt/1
  Rate Transition/1 -> Demux/1

== system COM_ViconController_x4morf_quat/GUMSTIX/Control Mix/Omega_ref 2 PWM_ref ==
  Omega_ref : Inport
  Bias : Bias  Bias=b_PWM
  Gain : Gain  Gain=a_PWM
  PWM_ref : Outport
  wires:
  Gain/1 -> Bias/1
  Bias/1 -> PWM_ref/1
  Omega_ref/1 -> Gain/1

== system COM_ViconController_x4morf_quat/GUMSTIX/ESTIMATOR/Complementary Filter Quaternion gyro, acc, vicon GUMSTIX ==
  gyro : Inport
  acc : Inport  Port=2
  Vicon_Quaternion : Inport  Port=3
  k_a : Inport  Port=4
  k_v : Inport  Port=5
  k_b : Inport  Port=6
  Attitude_Est : MATLAB Function  TreatAsAtomicUnit=on
  Bias : Delay  DelayLength=1  InitialCondition=b0_param  SampleTime=Ts_param
  Constant1 : Constant  Value=Ts_param  OutDataTypeStr=Inherit: Inherit via back propagation
  Constant7 : Constant  Value=acc_ref_param  VectorParams1D=off  OutDataTypeStr=Inherit: Inherit via back propagation
  Quaternion : Delay  DelayLength=1  InitialCondition=Q0_param  SampleTime=Ts_param
  b_hat [rad/sec] : Outport
  Q_hat : Outport  Port=2
  Omega_hat [rad/sec] : Outport  Port=3
  wires:
  Attitude_Est/1(Q_hat) -> Q_hat/1, Quaternion/1
  Attitude_Est/2(b_hat) -> Bias/1, b_hat [rad/sec]/1
  Constant1/1 -> Attitude_Est/6(dt)
  Bias/1 -> Attitude_Est/2(b_hat_prec)
  Quaternion/1 -> Attitude_Est/1(Q_hat_prec)
  Attitude_Est/3(Omega_hat) -> Omega_hat [rad/sec]/1
  acc/1 -> Attitude_Est/4(acc_imu)
  gyro/1 -> Attitude_Est/3(gyro_imu)
  Constant7/1 -> Attitude_Est/10(acc_ref)
  Vicon_Quaternion/1 -> Attitude_Est/5(Q_Vicon)
  k_a/1 -> Attitude_Est/7(k_a)
  k_v/1 -> Attitude_Est/8(k_v)
  k_b/1 -> Attitude_Est/9(k_b)

== system COM_ViconController_x4morf_quat/GUMSTIX/ESTIMATOR/Unbias Sensors ==
  Sensors : Inport
  Bias : Bias  Bias=-BiasAcc
  Constant : Constant  Value=single(Tacc)
  Demux2 : Demux  Outputs=[3 3]
  Product : Product  Multiplication=Matrix(*)  RndMeth=Zero
  int16_2_g : Gain  Gain=MPU6050.acc.int16_2_g  OutDataTypeStr=Inherit: Same as input
  int16_2_rad : Gain  Gain=MPU6050.gyr.int16_2_rad  OutDataTypeStr=Inherit: Same as input
  RAW_Gyro : Outport
  Unbiased_Acc : Outport  Port=2
  RAW_Acc : Outport  Port=3
  wires:
  Sensors/1 -> Demux2/1
  int16_2_g/1 -> RAW_Acc/1, Bias/1
  Demux2/1 -> int16_2_rad/1
  int16_2_rad/1 -> RAW_Gyro/1
  Demux2/2 -> int16_2_g/1
  Bias/1 -> Product/2
  Constant/1 -> Product/1
  Product/1 -> Unbiased_Acc/1

== system COM_ViconController_x4morf_quat/GUMSTIX/Manual_Controller/RX Angles Ref  Generator ==
  Roll_RX : Inport
  Pitch_RX : Inport  Port=2
  Yaw_RX : Inport  Port=3
  Throttle_RX : Inport  Port=4
  Rescale Pitch : Subsystem  mask{MinInput=1000, MaxInput=2000, DeadZone=10, MinOutput=-20*pi/180, MaxOutput=20*pi/180, G_Scale=0, BiasScale=0}
      mask prompts: MinInput "Minimum Input"; MaxInput "Maximum Input"; DeadZone "Dead Zone"; MinOutput "Minimum Output"; MaxOutput "Maximum Output"; BiasScale "Bias_Scale"
      mask init:
      | Gscale = (MaxOutput-MinOutput)/(MaxInput-MinInput-2*DeadZone);
      | Bias_Scale = MinInput+(MaxInput-MinInput)/2;
  Rescale Roll : Subsystem  mask{MinInput=1000, MaxInput=2000, DeadZone=10, MinOutput=-20*pi/180, MaxOutput=20*pi/180, G_Scale=0, BiasScale=0}
      mask prompts: MinInput "Minimum Input"; MaxInput "Maximum Input"; DeadZone "Dead Zone"; MinOutput "Minimum Output"; MaxOutput "Maximum Output"; BiasScale "Bias_Scale"
      mask init:
      | Gscale = (MaxOutput-MinOutput)/(MaxInput-MinInput-2*DeadZone);
      | Bias_Scale = MinInput+(MaxInput-MinInput)/2;
  Rescale Yaw : Subsystem  mask{MinInput=1000, MaxInput=2000, DeadZone=10, MinOutput=-30*pi/180, MaxOutput=30*pi/180, G_Scale=0, BiasScale=0}
      mask prompts: MinInput "Minimum Input"; MaxInput "Maximum Input"; DeadZone "Dead Zone"; MinOutput "Minimum Output"; MaxOutput "Maximum Output"; BiasScale "Bias_Scale"
      mask init:
      | Gscale = (MaxOutput-MinOutput)/(MaxInput-MinInput-2*DeadZone);
      | Bias_Scale = MinInput+(MaxInput-MinInput)/2;
  Rescale2 Throttle : Subsystem  mask{MinInput=1000, MaxInput=2000, MinOutput=0*m*g, MaxOutput=1.3*m*g, G_Scale=0}
      mask prompts: MinInput "Minimum Input"; MaxInput "Maximum Input"; MinOutput "Minimum Output"; MaxOutput "Maximum Output"
      mask init:
      | Gscale = (MaxOutput-MinOutput)/(MaxInput-MinInput);
  Roll_ref : Outport
  Pitch_ref : Outport  Port=2
  Yaw_ref : Outport  Port=3
  Throttle_ref : Outport  Port=4
  wires:
  Roll_RX/1 -> Rescale Roll/1(In)
  Pitch_RX/1 -> Rescale Pitch/1(In)
  Yaw_RX/1 -> Rescale Yaw/1(In)
  Rescale Roll/1(Out) -> Roll_ref/1
  Rescale Pitch/1(Out) -> Pitch_ref/1
  Rescale Yaw/1(Out) -> Yaw_ref/1
  Throttle_RX/1 -> Rescale2 Throttle/1(In)
  Rescale2 Throttle/1(Out) -> Throttle_ref/1

== system COM_ViconController_x4morf_quat/GUMSTIX/Positioning Mode/ClosedLoop Position SetPoint Generator ==
  WandMode : Inport
  X_ref : Inport  Port=2
  X0 : Inport  Port=3
  3 order discrete filter Trep1 : Subsystem  mask{Tau=[3/6 3/6 5/6]', Ts_Filter=1/100, Xmax=PositionMax, Xmin=PositionMin, Smax=SpeedMax, Smin=SpeedMin, Amax=AccMax, Amin=AccMin}
      mask prompts: Ts_Filter "Ts"; Xmax "Pos max"; Xmin "Pos min"; Smax "Speed max"; Smin "Speed min"; Amax "Acc max"; Amin "Acc min"
  3 order discrete filter Trep2 : Subsystem  mask{Tau=1/6, Ts_Filter=1/100, Xmax=PositionMax, Xmin=PositionMin, Smax=SpeedMax, Smin=SpeedMin, Amax=AccMax, Amin=AccMin}
      mask prompts: Ts_Filter "Ts"; Xmax "Pos max"; Xmin "Pos min"; Smax "Speed max"; Smin "Speed min"; Amax "Acc max"; Amin "Acc min"
  A_FF : MultiPortSwitch  DataPortOrder=Zero-based contiguous  Inputs=2  zeroidx=on
  Gyo Acc3 : Mux
  S_FF : MultiPortSwitch  DataPortOrder=Zero-based contiguous  Inputs=2  zeroidx=on
  X_FF : MultiPortSwitch  DataPortOrder=Zero-based contiguous  Inputs=2  zeroidx=on
  udp_received_from_gumstix demux1 : Demux  Outputs=[3 1]
  X_ref_FF : Outport
  wires:
  WandMode/1 -> X_FF/1, S_FF/1, A_FF/1
  3 order discrete filter Trep2/1(X_ref) -> X_FF/3
  3 order discrete filter Trep2/3(A_ref) -> A_FF/3
  3 order discrete filter Trep2/2(S_ref) -> S_FF/3
  S_FF/1 -> Gyo Acc3/2
  [X_ref] -> 3 order discrete filter Trep2/1(Ref), 3 order discrete filter Trep1/1(Ref)
  A_FF/1 -> Gyo Acc3/3
  3 order discrete filter Trep1/1(X_ref) -> X_FF/2
  3 order discrete filter Trep1/2(S_ref) -> S_FF/2
  3 order discrete filter Trep1/3(A_ref) -> A_FF/2
  X0/1 -> 3 order discrete filter Trep2/2(X0), 3 order discrete filter Trep1/2(X0)
  udp_received_from_gumstix demux1/1 -> [X_ref]
  udp_received_from_gumstix demux1/2 -> [Psi_ref]
  X_ref/1 -> udp_received_from_gumstix demux1/1
  X_FF/1 -> Gyo Acc3/1
  Gyo Acc3/1 -> X_ref_FF/1
  [Psi_ref] -> Gyo Acc3/4

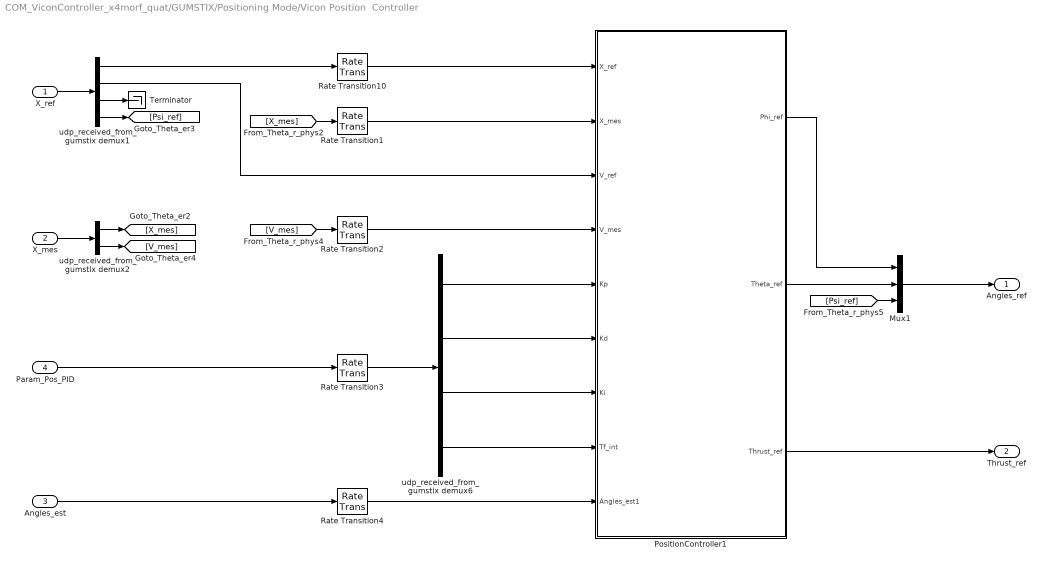
== system COM_ViconController_x4morf_quat/GUMSTIX/Positioning Mode/Vicon Position  Controller ==
  X_ref : Inport
  X_mes : Inport  Port=2
  Angles_est : Inport  Port=3
  Param_Pos_PID : Inport  Port=4
  Mux1 : Mux  Inputs=[1 1 1]
  PositionController1 : Subsystem
  Rate Transition{1..4,10} (5 alike) : RateTransition  OutPortSampleTime=Ts_PositionLoop
  Terminator : Terminator
  udp_received_from_gumstix demux1 : Demux  Outputs=[3 3 3 1]
  udp_received_from_gumstix demux2 : Demux  Outputs=[3 3]
  udp_received_from_gumstix demux6 : Demux  Outputs=[3 3 3 3]
  Angles_ref : Outport  InitialOutput=eye(3, 3)
  Thrust_ref : Outport  Port=2  InitialOutput=0
  wires:
  Mux1/1 -> Angles_ref/1
  PositionController1/3(Thrust_ref) -> Thrust_ref/1
  X_ref/1 -> udp_received_from_gumstix demux1/1
  udp_received_from_gumstix demux1/1 -> Rate Transition10/1
  [X_mes] -> Rate Transition1/1
  [V_mes] -> Rate Transition2/1
  Angles_est/1 -> Rate Transition4/1
  Param_Pos_PID/1 -> Rate Transition3/1
  X_mes/1 -> udp_received_from_gumstix demux2/1
  udp_received_from_gumstix demux2/1 -> [X_mes]
  udp_received_from_gumstix demux2/2 -> [V_mes]
  udp_received_from_gumstix demux1/4 -> [Psi_ref]
  PositionController1/1(Phi_ref) -> Mux1/1
  PositionController1/2(Theta_ref) -> Mux1/2
  udp_received_from_gumstix demux1/2 -> PositionController1/3(V_ref)
  Rate Transition10/1 -> PositionController1/1(X_ref)
  Rate Transition1/1 -> PositionController1/2(X_mes)
  Rate Transition2/1 -> PositionController1/4(V_mes)
  Rate Transition3/1 -> udp_received_from_gumstix demux6/1
  Rate Transition4/1 -> PositionController1/9(Angles_est1)
  [Psi_ref] -> Mux1/3
  udp_received_from_gumstix demux6/1 -> PositionController1/5(Kp)
  udp_received_from_gumstix demux6/2 -> PositionController1/6(Kd)
  udp_received_from_gumstix demux6/3 -> PositionController1/7(Ki)
  udp_received_from_gumstix demux6/4 -> PositionController1/8(Tf_int)
  udp_received_from_gumstix demux1/3 -> Terminator/1

== system COM_ViconController_x4morf_quat/GUMSTIX/Torques  Disturbances/Triggered Subsystem ==
  TorquesDist Mag : Inport
  Dt : Inport  Port=2
  Enable : EnablePort  StatesWhenEnabling=reset
  Constant : Constant  OutDataTypeStr=single
  Discrete-Time Integrator : DiscreteIntegrator  SampleTime=-1  ICPrevOutput=DiscIntNeverNeededParam  ICPrevScaledInput=DiscIntNeverNeededParam
  MATLAB Function : MATLAB Function  TreatAsAtomicUnit=on
  DisturbTorques : Outport  InitialOutput=[0 0 0]
  wires:
  TorquesDist Mag/1 -> MATLAB Function/1(TorquesDistMag)
  Constant/1 -> Discrete-Time Integrator/1
  Discrete-Time Integrator/1 -> MATLAB Function/2(Time)
  Dt/1 -> MATLAB Function/3(Dt)
  MATLAB Function/1(TorquesDist) -> DisturbTorques/1
